simulink model "finale"  (R2016a)
settings: Solver=FixedStepAuto  SolverMode=SingleTasking  StartTime=0.0  StopTime=800000  RelTol=1e-3
undefined symbols (not defined in the file or in its folder): Cb, Ch, Cw, Cwym, Kext, Kh, Kw, Mb, Mco, Mh, Mm, ro, T0
libraries: simulink x3
settings Model: Creator=Konrad  LastModifiedBy=dorot
settings OptimizationCC: DefaultParameterBehavior=Inlined  UseDivisionForNetSlopeComputation=on  UseFloatMulNetSlope=on  InlineInvariantSignals=on  PassReuseOutputArgsAs=Individual arguments  ZeroExternalMemoryAtStartup=off  ZeroInternalMemoryAtStartup=off  NoFixptDivByZeroProtection=on  EfficientFloat2IntCast=on  OptimizeModelRefInitCode=on  LifeSpan=1
settings DebuggingCC: SFUnexpectedBacktrackingDiag=error  SFNoUnconditionalDefaultTransitionDiag=error
settings SFSimCC: SimUseLocalCustomCode=on
settings RTWCC: SystemTargetFile=ert.tlc  TemplateMakefile=ert_default_tmf  GenerateReport=on  RTWUseLocalCustomCode=on  IncludeHyperlinkInReport=on  LaunchReport=on  GenerateTraceInfo=on  GenerateTraceReport=on  GenerateTraceReportSl=on  GenerateTraceReportSf=on  GenerateTraceReportEml=on  GenerateCodeMetricsReport=on
settings CodeAppCC: ForceParamTrailComments=on  IgnoreCustomStorageClasses=off  OperatorAnnotations=on  SimulinkDataObjDesc=on  SFDataObjDesc=on  MATLABFcnDesc=on  CustomSymbolStrGlobalVar=rt$N$M  CustomSymbolStrType=$N$M  CustomSymbolStrFcn=$N$M$F  CustomSymbolStrMacro=$N$M  InsertBlockDesc=on  MATLABSourceComments=on
settings ERTTargetCC: GenerateSampleERTMain=on  IncludeMdlTerminateFcn=off  CombineSignalStateStructs=on  SupportAbsoluteTime=off  SupportComplex=off  SupportContinuousTime=on  InlinedParameterPlacement=NonHierarchical  ERTCustomFileTemplate=example_file_process.tlc  ERTFilePackagingFormat=CompactWithDataFile
settings ConfigComp: CovMetricSettings=dwe  CovHtmlReporting=off  CovSaveCumulativeToWorkspaceVar=off  CovSaveSingleToWorkspaceVar=off  CovExternalEMLEnable=on

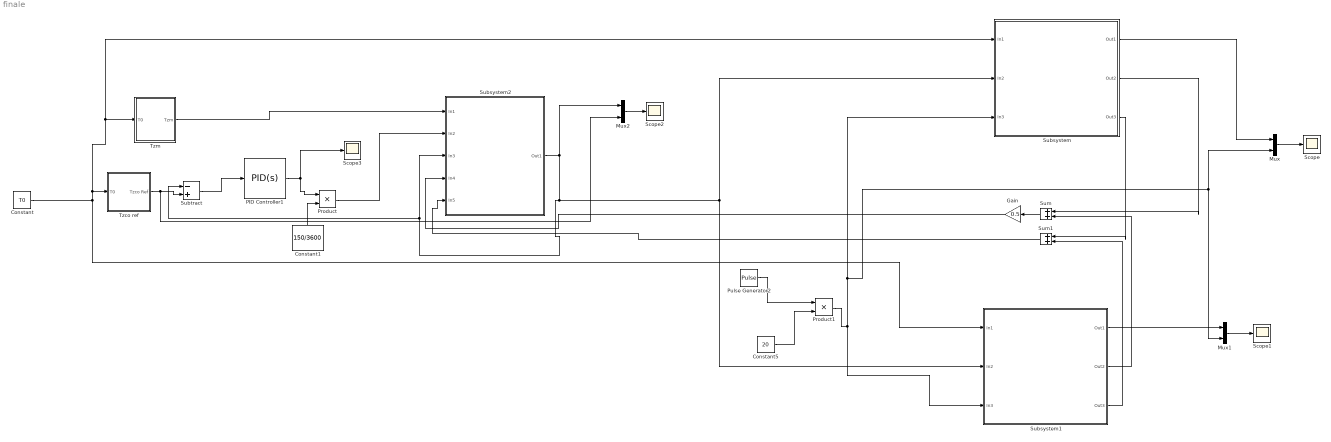
== system finale ==
  Constant : Constant  Value=T0
  Constant1 : Constant  Value=150/3600
  Constant5 : Constant  Value=20
  Gain : Gain  Gain=0.5
  Mux : Mux  Inputs=2
  Mux1 : Mux  Inputs=2
  Mux2 : Mux  Inputs=2
  PID Controller1 : simulink/Continuous/PID Controller  Controller=PID  TimeDomain=Continuous-time  SampleTime=-1  IntegratorMethod=Forward Euler  FilterMethod=Forward Euler  Form=Ideal  UseFilter=on  ControllerParametersSource=internal  P=1  I=0  D=0  N=100  InitialConditionSource=internal  InitialConditionForIntegrator=0  InitialConditionForFilter=0  ExternalReset=none  LimitOutput=on  UpperSaturationLimit=1  LowerSaturationLimit=0  LinearizeAsGain=on  AntiWindupMode=none  Kb=1  TrackingMode=off  Kt=1  PParamMin=[]  PParamMax=[]  IParamMin=[]  IParamMax=[]  DParamMin=[]  DParamMax=[]  NParamMin=[]  NParamMax=[]  KbParamMin=[]  KbParamMax=[]  KtParamMin=[]  KtParamMax=[]  POutMin=[]  POutMax=[]  IOutMin=[]  IOutMax=[]  DOutMin=[]  DOutMax=[]  NOutMin=[]  NOutMax=[]  KbOutMin=[]  KbOutMax=[]  KtOutMin=[]  KtOutMax=[]  IntegratorOutMin=[]  IntegratorOutMax=[]  FilterOutMin=[]  FilterOutMax=[]  SumOutMin=[]  SumOutMax=[]  SumI1OutMin=[]  SumI1OutMax=[]  SumI2OutMin=[]  SumI2OutMax=[]  SumI3OutMin=[]  SumI3OutMax=[]  SumDOutMin=[]  SumDOutMax=[]  SaturationOutMin=[]  SaturationOutMax=[]  IntegratorContinuousStateAttributes=''  IntegratorStateMustResolveToSignalObject=off  IntegratorRTWStateStorageClass=Auto  FilterContinuousStateAttributes=''  FilterStateMustResolveToSignalObject=off  FilterRTWStateStorageClass=Auto  DifferentiatorICPrevScaledInput=0  DifferentiatorOutMin=[]  DifferentiatorOutMax=[]
  Product : Product
  Product1 : Product
  Pulse Generator2 : DiscretePulseGenerator  PulseType=Time based  Amplitude=10  Period=80000/3  PulseWidth=5/7*100
  Scope{,1..3} (4 alike) : Scope
  Subsystem : Subsystem
  Subsystem1 : Subsystem
  Subsystem2 : Subsystem
  Subtract : Sum  Inputs=-+
  Sum : Sum  Inputs=|++
  Sum1 : Sum  Inputs=|++
  "Tzco ref " : Subsystem
  Tzm : Subsystem
  wires:
  Subtract/1 -> PID Controller1/1
  PID Controller1/1 -> Product/1, Scope3/1
  Constant1/1 -> Product/2
  "Tzco ref "/1("Tzco Ref ") -> Mux2/2, Subtract/2
  Sum/1 -> Gain/1
  Constant/1 -> Subsystem1/1(In1), Subsystem/1(In1), Tzm/1(T0), "Tzco ref "/1("T0 ")
  Mux/1 -> Scope/1
  Product1/1 -> Subsystem/3(In3), Mux1/2, Mux/2, Subsystem1/3(In3)
  Subsystem/1(Out1) -> Mux/1
  Subsystem/2(Out2) -> Sum/1
  Subsystem/3(Out3) -> Sum1/1
  Subsystem1/2(Out2) -> Sum/2
  Subsystem1/3(Out3) -> Sum1/2
  Tzm/1("Tzm ") -> Subsystem2/1(In1)
  Product/1 -> Subsystem2/2(In2)
  Gain/1 -> Subsystem2/4(In4)
  Sum1/1 -> Subsystem2/5(In5)
  Mux1/1 -> Scope1/1
  Subsystem1/1(Out1) -> Mux1/1
  Mux2/1 -> Scope2/1
  Subsystem2/1(Out1) -> Subsystem2/3(In3), Subtract/1, Subsystem1/2(In2), Subsystem/2(In2), Mux2/1
  Constant5/1 -> Product1/2
  Pulse Generator2/1 -> Product1/1

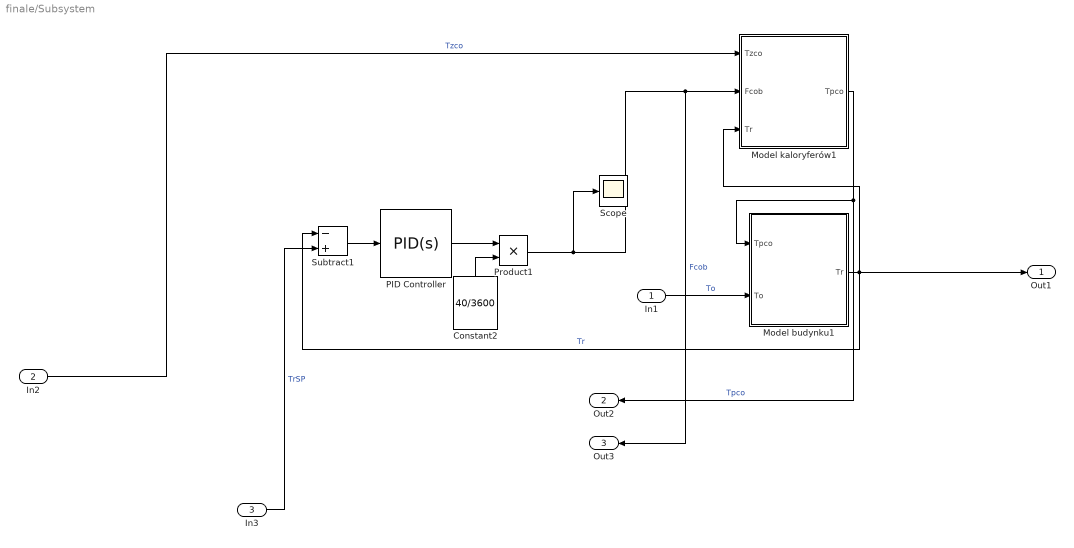
== system finale/Subsystem ==
  In1 : Inport
  In2 : Inport  Port=2
  In3 : Inport  Port=3
  Constant2 : Constant  Value=40/3600
  Model budynku1 : Subsystem
  Model kaloryferów1 : Subsystem
  PID Controller : simulink/Continuous/PID Controller  Controller=PID  TimeDomain=Continuous-time  SampleTime=-1  IntegratorMethod=Forward Euler  FilterMethod=Forward Euler  Form=Ideal  UseFilter=on  ControllerParametersSource=internal  P=1  I=0  D=0  N=100  InitialConditionSource=internal  InitialConditionForIntegrator=0  InitialConditionForFilter=0  ExternalReset=none  LimitOutput=on  UpperSaturationLimit=1  LowerSaturationLimit=0  LinearizeAsGain=on  AntiWindupMode=none  Kb=1  TrackingMode=off  Kt=1  PParamMin=[]  PParamMax=[]  IParamMin=[]  IParamMax=[]  DParamMin=[]  DParamMax=[]  NParamMin=[]  NParamMax=[]  KbParamMin=[]  KbParamMax=[]  KtParamMin=[]  KtParamMax=[]  POutMin=[]  POutMax=[]  IOutMin=[]  IOutMax=[]  DOutMin=[]  DOutMax=[]  NOutMin=[]  NOutMax=[]  KbOutMin=[]  KbOutMax=[]  KtOutMin=[]  KtOutMax=[]  IntegratorOutMin=[]  IntegratorOutMax=[]  FilterOutMin=[]  FilterOutMax=[]  SumOutMin=[]  SumOutMax=[]  SumI1OutMin=[]  SumI1OutMax=[]  SumI2OutMin=[]  SumI2OutMax=[]  SumI3OutMin=[]  SumI3OutMax=[]  SumDOutMin=[]  SumDOutMax=[]  SaturationOutMin=[]  SaturationOutMax=[]  IntegratorContinuousStateAttributes=''  IntegratorStateMustResolveToSignalObject=off  IntegratorRTWStateStorageClass=Auto  FilterContinuousStateAttributes=''  FilterStateMustResolveToSignalObject=off  FilterRTWStateStorageClass=Auto  DifferentiatorICPrevScaledInput=0  DifferentiatorOutMin=[]  DifferentiatorOutMax=[]
  Product1 : Product
  Scope : Scope
  Subtract1 : Sum  Inputs=-+
  Out1 : Outport
  Out2 : Outport  Port=2
  Out3 : Outport  Port=3
  wires:
  In3/1 -> Subtract1/2  "TrSP"
  Model kaloryferów1/1("Tpco ") -> Out2/1, Model budynku1/1(Tpco)  "Tpco"
  Product1/1 -> Scope/1, Out3/1, Model kaloryferów1/2(Fcob)  "Fcob"
  Model budynku1/1(Tr) -> Model kaloryferów1/3(Tr), Out1/1, Subtract1/1  "Tr"
  In1/1 -> Model budynku1/2(To)  "To"
  PID Controller/1 -> Product1/1
  Subtract1/1 -> PID Controller/1
  Constant2/1 -> Product1/2
  In2/1 -> Model kaloryferów1/1(Tzco)  "Tzco"

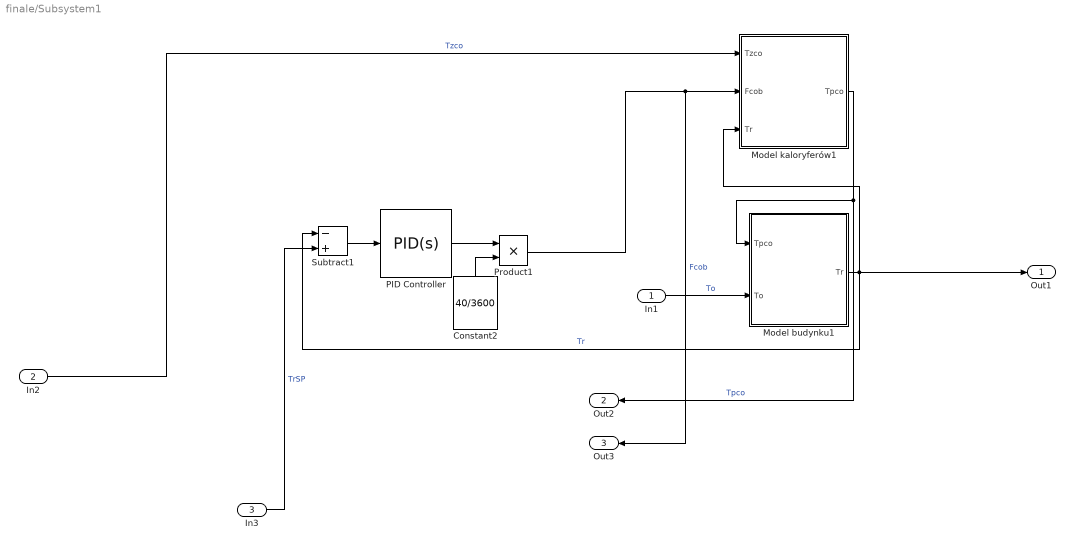
== system finale/Subsystem1 ==
  In1 : Inport
  In2 : Inport  Port=2
  In3 : Inport  Port=3
  Constant2 : Constant  Value=40/3600
  Model budynku1 : Subsystem
  Model kaloryferów1 : Subsystem
  PID Controller : simulink/Continuous/PID Controller  Controller=PID  TimeDomain=Continuous-time  SampleTime=-1  IntegratorMethod=Forward Euler  FilterMethod=Forward Euler  Form=Ideal  UseFilter=on  ControllerParametersSource=internal  P=1  I=0  D=0  N=100  InitialConditionSource=internal  InitialConditionForIntegrator=0  InitialConditionForFilter=0  ExternalReset=none  LimitOutput=on  UpperSaturationLimit=1  LowerSaturationLimit=0  LinearizeAsGain=on  AntiWindupMode=none  Kb=1  TrackingMode=off  Kt=1  PParamMin=[]  PParamMax=[]  IParamMin=[]  IParamMax=[]  DParamMin=[]  DParamMax=[]  NParamMin=[]  NParamMax=[]  KbParamMin=[]  KbParamMax=[]  KtParamMin=[]  KtParamMax=[]  POutMin=[]  POutMax=[]  IOutMin=[]  IOutMax=[]  DOutMin=[]  DOutMax=[]  NOutMin=[]  NOutMax=[]  KbOutMin=[]  KbOutMax=[]  KtOutMin=[]  KtOutMax=[]  IntegratorOutMin=[]  IntegratorOutMax=[]  FilterOutMin=[]  FilterOutMax=[]  SumOutMin=[]  SumOutMax=[]  SumI1OutMin=[]  SumI1OutMax=[]  SumI2OutMin=[]  SumI2OutMax=[]  SumI3OutMin=[]  SumI3OutMax=[]  SumDOutMin=[]  SumDOutMax=[]  SaturationOutMin=[]  SaturationOutMax=[]  IntegratorContinuousStateAttributes=''  IntegratorStateMustResolveToSignalObject=off  IntegratorRTWStateStorageClass=Auto  FilterContinuousStateAttributes=''  FilterStateMustResolveToSignalObject=off  FilterRTWStateStorageClass=Auto  DifferentiatorICPrevScaledInput=0  DifferentiatorOutMin=[]  DifferentiatorOutMax=[]
  Product1 : Product
  Subtract1 : Sum  Inputs=-+
  Out1 : Outport
  Out2 : Outport  Port=2
  Out3 : Outport  Port=3
  wires:
  In3/1 -> Subtract1/2  "TrSP"
  Model kaloryferów1/1("Tpco ") -> Out2/1, Model budynku1/1(Tpco)  "Tpco"
  Product1/1 -> Out3/1, Model kaloryferów1/2(Fcob)  "Fcob"
  Model budynku1/1(Tr) -> Model kaloryferów1/3(Tr), Out1/1, Subtract1/1  "Tr"
  In1/1 -> Model budynku1/2(To)  "To"
  PID Controller/1 -> Product1/1
  Subtract1/1 -> PID Controller/1
  Constant2/1 -> Product1/2
  In2/1 -> Model kaloryferów1/1(Tzco)  "Tzco"

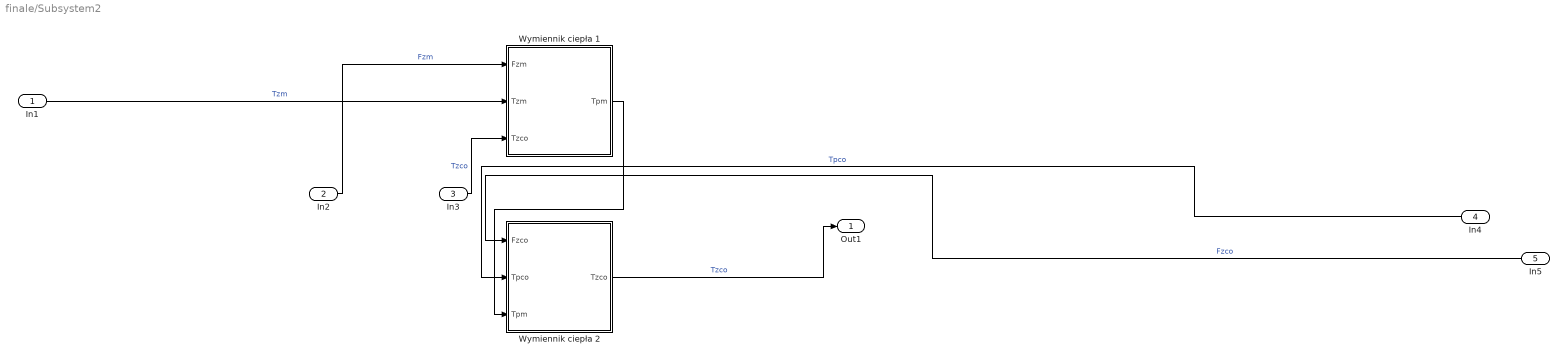
== system finale/Subsystem2 ==
  In1 : Inport
  In2 : Inport  Port=2
  In3 : Inport  Port=3
  In4 : Inport  Port=4
  In5 : Inport  Port=5
  "Wymiennik ciepła 1 " : Subsystem
  "Wymiennik ciepła 2 " : Subsystem
  Out1 : Outport
  wires:
  "Wymiennik ciepła 2 "/1(Tzco) -> Out1/1  "Tzco"
  "Wymiennik ciepła 1 "/1(Tpm) -> "Wymiennik ciepła 2 "/3(Tpm)
  In1/1 -> "Wymiennik ciepła 1 "/2(Tzm)  "Tzm"
  In4/1 -> "Wymiennik ciepła 2 "/2("Tpco ")  "Tpco"
  In3/1 -> "Wymiennik ciepła 1 "/3(Tzco)  "Tzco"
  In2/1 -> "Wymiennik ciepła 1 "/1("Fzm ")  "Fzm"
  In5/1 -> "Wymiennik ciepła 2 "/1("Fzco ")  "Fzco"

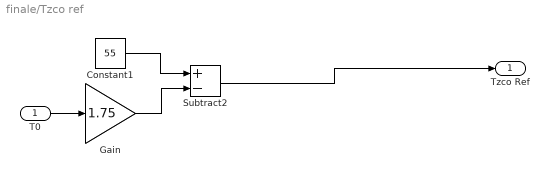
== system finale/Tzco ref  ==
  "T0 " : Inport
  Constant1 : Constant  Value=55
  Gain : Gain  Gain=1.75
  Subtract2 : Sum  Inputs=+-
  "Tzco Ref " : Outport
  wires:
  "T0 "/1 -> Gain/1
  Constant1/1 -> Subtract2/1
  Gain/1 -> Subtract2/2
  Subtract2/1 -> "Tzco Ref "/1

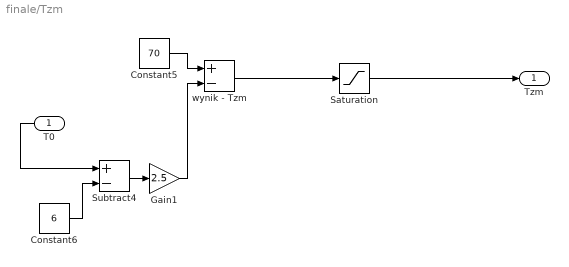
== system finale/Tzm ==
  T0 : Inport
  Constant5 : Constant  Value=70
  Constant6 : Constant  Value=6
  Gain1 : Gain  Gain=2.5
  Saturation : Saturate  UpperLimit=135  LowerLimit=70
  Subtract4 : Sum  Inputs=+-
  "wynik - Tzm " : Sum  Inputs=+-
  "Tzm " : Outport
  wires:
  Constant6/1 -> Subtract4/2
  Constant5/1 -> "wynik - Tzm "/1
  Subtract4/1 -> Gain1/1
  Gain1/1 -> "wynik - Tzm "/2
  "wynik - Tzm "/1 -> Saturation/1
  T0/1 -> Subtract4/1
  Saturation/1 -> "Tzm "/1

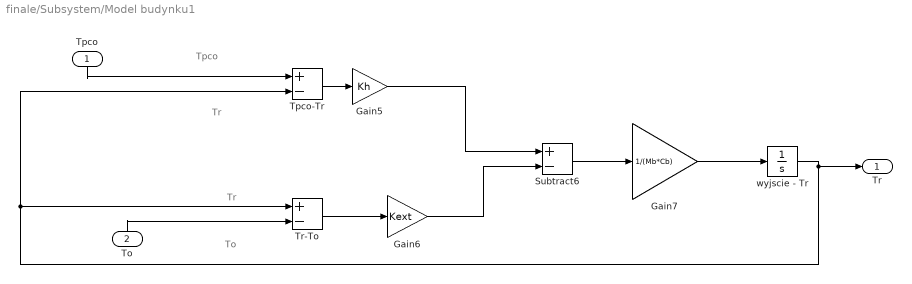
== system finale/Subsystem/Model budynku1 ==
  note: To
  note: Tr
  note: Tr
  note: Tpco
  Tpco : Inport
  To : Inport  Port=2
  Gain5 : Gain  Gain=Kh
  Gain6 : Gain  Gain=Kext
  Gain7 : Gain  Gain=1/(Mb*Cb)
  Subtract6 : Sum  Inputs=+-
  Tpco-Tr : Sum  Inputs=+-
  Tr-To : Sum  Inputs=+-
  wyjscie - Tr : Integrator
  Tr : Outport
  wires:
  To/1 -> Tr-To/2
  Gain6/1 -> Subtract6/2
  Gain7/1 -> wyjscie - Tr/1
  Tpco/1 -> Tpco-Tr/1
  Subtract6/1 -> Gain7/1
  wyjscie - Tr/1 -> Tr/1, Tr-To/1, Tpco-Tr/2
  Tpco-Tr/1 -> Gain5/1
  Tr-To/1 -> Gain6/1
  Gain5/1 -> Subtract6/1

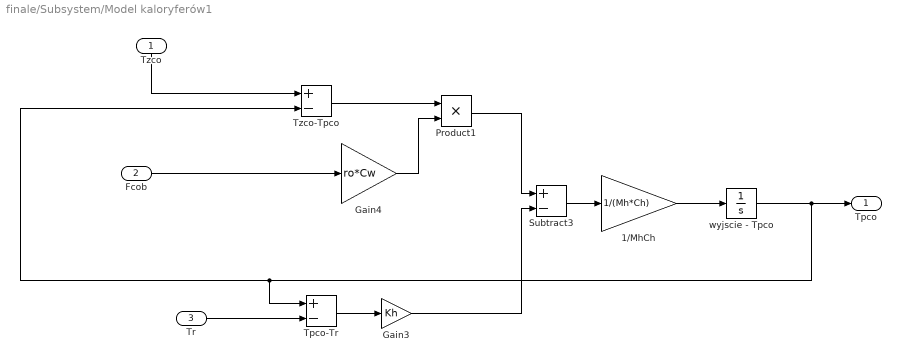
== system finale/Subsystem/Model kaloryferów1 ==
  Tzco : Inport
  Fcob : Inport  Port=2
  Tr : Inport  Port=3
  1/MhCh : Gain  Gain=1/(Mh*Ch)
  Gain3 : Gain  Gain=Kh
  Gain4 : Gain  Gain=ro*Cw
  Product1 : Product
  Subtract3 : Sum  Inputs=+-
  Tpco-Tr : Sum  Inputs=+-
  Tzco-Tpco : Sum  Inputs=+-
  wyjscie - Tpco : Integrator
  "Tpco " : Outport
  wires:
  Tpco-Tr/1 -> Gain3/1
  Subtract3/1 -> 1/MhCh/1
  Fcob/1 -> Gain4/1
  wyjscie - Tpco/1 -> "Tpco "/1, Tpco-Tr/1, Tzco-Tpco/2
  Tzco-Tpco/1 -> Product1/1
  Tzco/1 -> Tzco-Tpco/1
  Product1/1 -> Subtract3/1
  Gain4/1 -> Product1/2
  Gain3/1 -> Subtract3/2
  Tr/1 -> Tpco-Tr/2
  1/MhCh/1 -> wyjscie - Tpco/1

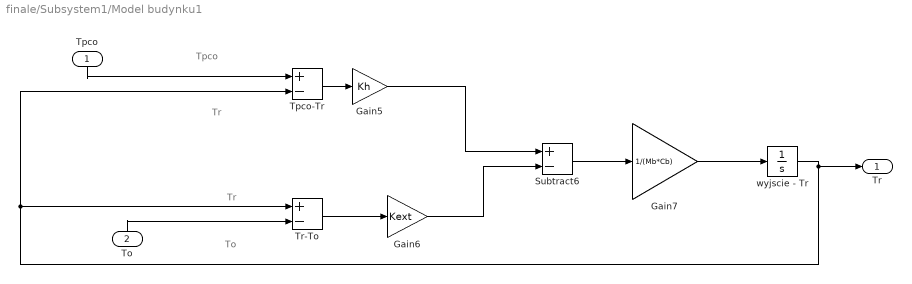
== system finale/Subsystem1/Model budynku1 ==
  note: To
  note: Tr
  note: Tr
  note: Tpco
  Tpco : Inport
  To : Inport  Port=2
  Gain5 : Gain  Gain=Kh
  Gain6 : Gain  Gain=Kext
  Gain7 : Gain  Gain=1/(Mb*Cb)
  Subtract6 : Sum  Inputs=+-
  Tpco-Tr : Sum  Inputs=+-
  Tr-To : Sum  Inputs=+-
  wyjscie - Tr : Integrator
  Tr : Outport
  wires:
  To/1 -> Tr-To/2
  Gain6/1 -> Subtract6/2
  Gain7/1 -> wyjscie - Tr/1
  Tpco/1 -> Tpco-Tr/1
  Subtract6/1 -> Gain7/1
  wyjscie - Tr/1 -> Tr/1, Tr-To/1, Tpco-Tr/2
  Tpco-Tr/1 -> Gain5/1
  Tr-To/1 -> Gain6/1
  Gain5/1 -> Subtract6/1

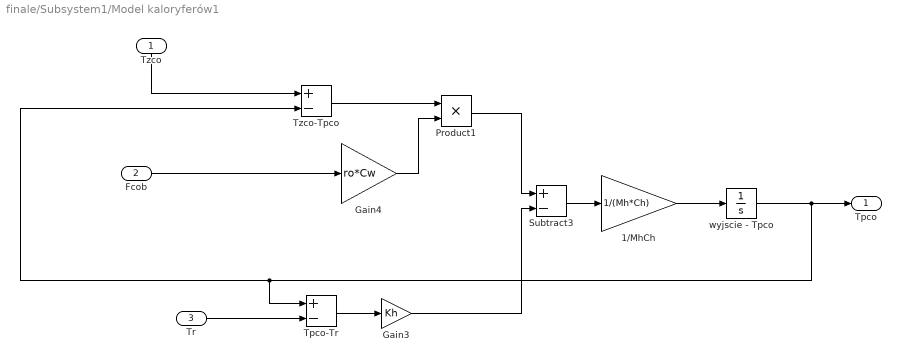
== system finale/Subsystem1/Model kaloryferów1 ==
  Tzco : Inport
  Fcob : Inport  Port=2
  Tr : Inport  Port=3
  1/MhCh : Gain  Gain=1/(Mh*Ch)
  Gain3 : Gain  Gain=Kh
  Gain4 : Gain  Gain=ro*Cw
  Product1 : Product
  Subtract3 : Sum  Inputs=+-
  Tpco-Tr : Sum  Inputs=+-
  Tzco-Tpco : Sum  Inputs=+-
  wyjscie - Tpco : Integrator
  "Tpco " : Outport
  wires:
  Tpco-Tr/1 -> Gain3/1
  Subtract3/1 -> 1/MhCh/1
  Fcob/1 -> Gain4/1
  wyjscie - Tpco/1 -> "Tpco "/1, Tpco-Tr/1, Tzco-Tpco/2
  Tzco-Tpco/1 -> Product1/1
  Tzco/1 -> Tzco-Tpco/1
  Product1/1 -> Subtract3/1
  Gain4/1 -> Product1/2
  Gain3/1 -> Subtract3/2
  Tr/1 -> Tpco-Tr/2
  1/MhCh/1 -> wyjscie - Tpco/1

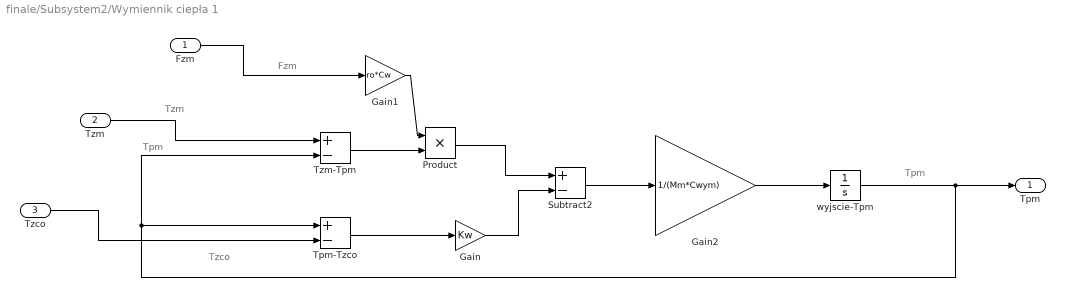
== system finale/Subsystem2/Wymiennik ciepła 1  ==
  note: Tpm
  note: Tzco
  note: Tpm
  note: Tzm
  note: Fzm
  "Fzm " : Inport
  Tzm : Inport  Port=2
  Tzco : Inport  Port=3
  Gain : Gain  Gain=Kw
  Gain1 : Gain  Gain=ro*Cw
  Gain2 : Gain  Gain=1/(Mm*Cwym)
  Product : Product
  Subtract2 : Sum  Inputs=+-
  Tpm-Tzco : Sum  Inputs=+-
  Tzm-Tpm : Sum  Inputs=+-
  wyjscie-Tpm : Integrator
  Tpm : Outport
  wires:
  Tpm-Tzco/1 -> Gain/1
  Gain/1 -> Subtract2/2
  Tzm-Tpm/1 -> Product/2
  Tzm/1 -> Tzm-Tpm/1
  "Fzm "/1 -> Gain1/1
  Subtract2/1 -> Gain2/1
  Tzco/1 -> Tpm-Tzco/2
  wyjscie-Tpm/1 -> Tpm/1, Tpm-Tzco/1, Tzm-Tpm/2
  Gain2/1 -> wyjscie-Tpm/1
  Gain1/1 -> Product/1
  Product/1 -> Subtract2/1

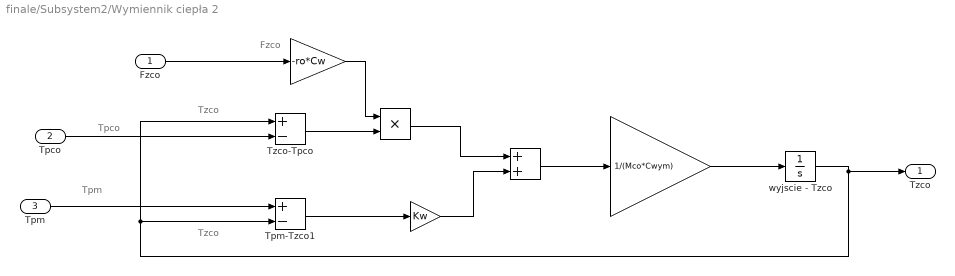
== system finale/Subsystem2/Wymiennik ciepła 2  ==
  note: Tpm
  note: Tzco
  note: Tpco
  note: Tzco
  note: Fzco
  "Fzco " : Inport
  "Tpco " : Inport  Port=2
  Tpm : Inport  Port=3
  " " : Gain  Gain=-ro*Cw
  "  " : Product
  "   " : Gain  Gain=Kw
  "    " : Sum
  "     " : Gain  Gain=1/(Mco*Cwym)
  Tpm-Tzco1 : Sum  Inputs=+-
  Tzco-Tpco : Sum  Inputs=+-
  "wyjscie - Tzco " : Integrator
  Tzco : Outport
  wires:
  "   "/1 -> "    "/2
  "Fzco "/1 -> " "/1
  Tpm-Tzco1/1 -> "   "/1
  Tzco-Tpco/1 -> "  "/2
  " "/1 -> "  "/1
  "     "/1 -> "wyjscie - Tzco "/1
  "Tpco "/1 -> Tzco-Tpco/2
  "    "/1 -> "     "/1
  "wyjscie - Tzco "/1 -> Tzco/1, Tzco-Tpco/1, Tpm-Tzco1/2
  Tpm/1 -> Tpm-Tzco1/1
  "  "/1 -> "    "/1
